simulink model "signal_pistolet"  (Simulink 7.9)
settings: Solver=ode45  StartTime=0.0  StopTime=Tsim  RelTol=1e-3
values from neighbouring files (symbols this model uses):
  Ampl = 5    [detection_tir (2014_06_05 20_25_39 UTC).m]
  F1 = 85005.9    [detection_tir (2014_06_05 20_25_39 UTC).m]
  F2 = 90000    [detection_tir (2014_06_05 20_25_39 UTC).m]
  F3 = 94986.8    [detection_tir (2014_06_05 20_25_39 UTC).m]
  F4 = 100000    [detection_tir (2014_06_05 20_25_39 UTC).m]
  F5 = 115015.9    [detection_tir (2014_06_05 20_25_39 UTC).m]
  F6 = 120000    [detection_tir (2014_06_05 20_25_39 UTC).m]
  Te = 1/Fe    (= 3.125e-06)    [detection_tir (2014_06_05 20_25_39 UTC).m]
settings Model: Creator=rprevost  LastModifiedBy=rprevost

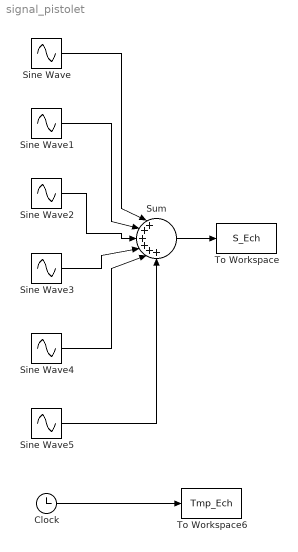
== system signal_pistolet ==
  Clock : Clock
  Sine Wave : Sin  Amplitude=Ampl  Frequency=F1*2*pi  SampleTime=0
  Sine Wave1 : Sin  Amplitude=Ampl  Frequency=F2*2*pi  SampleTime=0
  Sine Wave2 : Sin  Amplitude=Ampl  Frequency=F3*2*pi  SampleTime=0
  Sine Wave3 : Sin  Amplitude=Ampl  Frequency=F4*2*pi  SampleTime=0
  Sine Wave4 : Sin  Amplitude=Ampl  Frequency=F5*2*pi  SampleTime=0
  Sine Wave5 : Sin  Amplitude=Ampl  Frequency=F6*2*pi  SampleTime=0
  Sum : Sum  Inputs=|++++++
  To Workspace : ToWorkspace  VariableName=S_Ech  SampleTime=-1
  To Workspace6 : ToWorkspace  VariableName=Tmp_Ech  SampleTime=Te
  wires:
  Sine Wave/1 -> Sum/1
  Sine Wave1/1 -> Sum/2
  Sine Wave2/1 -> Sum/3
  Sine Wave3/1 -> Sum/4
  Sine Wave4/1 -> Sum/5
  Sine Wave5/1 -> Sum/6
  Clock/1 -> To Workspace6/1
  Sum/1 -> To Workspace/1
